simulink model "spwm_three_phase"  (R2020a)
settings: Solver=VariableStepAuto  StartTime=0.0  StopTime=3.0  RelTol=1e-3
values from neighbouring files (symbols this model uses):
  freq_rad = 2*pi*50    (= 314.159265359)    [three_phase_spwm.m]
  Gain = 2000    [three_phase_spwm.m]
  period = 2e-4    (= 0.0002)    [three_phase_spwm.m]
  phase_A = 0    [three_phase_spwm.m]
  phase_B = -2*pi/3    (= -2.09439510239)    [three_phase_spwm.m]
  phase_C = -4*pi/3    (= -4.18879020479)    [three_phase_spwm.m]
  pulse_width = 50    [three_phase_spwm.m]
  T_final_value = 1000    [three_phase_spwm.m]
  T_load_step_time = 1    [three_phase_spwm.m]
  Tz = 1/freq    (= 0.02)    [three_phase_spwm.m]
  Vamp = 1    [three_phase_spwm.m]
  VDC = 400    [three_phase_spwm.m]
  Vpulse = 10    [three_phase_spwm.m]
  Vref = (2/3)*VDC*0.9    (= 240)    [three_phase_spwm.m]
libraries: powerlib x5
settings Model: Creator=Junaed  LastModifiedBy=PC

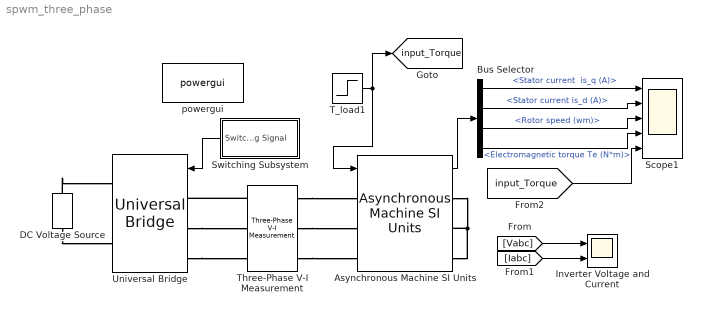
== system spwm_three_phase ==
  Asynchronous Machine SI Units : powerlib/Machines/Asynchronous Machine SI Units  RotorType=Wound  PresetModel=No  MechanicalLoad=Torque Tm  ShowDetailedParameters=on  ReferenceFrame=Rotor  Units=SI  MeasurementBus=off  NominalParameters=[1.845e+04 400 50]  Stator=[0.5968 0.0003495]  Rotor=[0.6258 0.005473]  Cage1=[0.4155 0.002066]  Cage2=[0.4168 0.0003495]  Lm=0.0354  Mechanical=[0.05 0.005879 2]  PolePairs=2  InitialConditions=[1 0 0 0 0 0 0 0]  SimulateSaturation=off  Saturation=[14.03593122, 27.81365428, 53.79336849, 72.68890987, 97.98006896, 148.6815601, 215.7428561, 302.9841135, 428.7778367 ; 230, 322, 414, 460, 506, 552, 598, 644, 690]  LoadFlowParameters=1492000  TsPowergui=0  TsBlock=-1  IterativeModel=Trapezoidal non iterative  IterativeDiscreteModel=Trapezoidal non iterative  Pmec=1.492e+006
  Bus Selector : BusSelector  OutputSignals="Stator measurements.Stator current  is_q (A),Stator measurements.Stator current is_d (A),Mechanical.Rotor speed (wm),Mechanical.Electromagnetic torque Te (N*m)"
  DC Voltage Source : powerlib/Electrical Sources/DC Voltage Source  Amplitude=VDC  Measurements=None
  Inverter Voltage and Current : Scope  NumInputPorts=2
  Scope1 : Scope  NumInputPorts=5
  Switching Subsystem : Subsystem
      settings: PortSchema="{\"entries\":[{\"content\":{\"sides\":[{\"content\":{\"connectorIds\":[\"Out1\"]},\"type\":\"ConnectorPlacement.EquallySpacedRectSide\",\"uuid\":\"666120e6-e3a6-4d41-8608-f47cc973ff78\"},{\"content\":{\"connectorIds\":[],\"side\":\"RIGHT\"},\"type\":\"ConnectorPlacement.EquallySpacedRectSide\",\"uuid\":\"51b09ffb-5a1b-4931-8ff6-f2d904303abf\"},{\"content\":{\"connectorIds\":[],\"side\":\"TOP\"},\"type\":\"ConnectorPlacement.EquallySpacedRectSide\",\"uuid\":\"d8637988-4995-4d87-a31f-ae42bffd7a57\"}]},\"type\":\"ConnectorPlacement.EquallySpacedConnector\",\"uuid\":\"019588fd-0135-4367-b5fb-8d28a8d71eb3\"}],\"packageUris\":[\"http://schema.mathworks.com/mf0/Connector/19700101\"],\"version\":\"1.0\"}"
  T_load1 : Step  Time=T_load_step_time  After=T_final_value  SampleTime=0
  Three-Phase V-I Measurement : powerlib/Measurements/Three-Phase V-I Measurement  VoltageMeasurement=phase-to-phase  SetLabelV=on  LabelV=Vabc  Vpu=off  VpuLL=off  CurrentMeasurement=yes  SetLabelI=on  LabelI=Iabc  Ipu=off  Pbase=100e6  Vbase=500e3  OutputType=Complex  PhasorSimulation=off  PSBequivalent=0
  Universal Bridge : powerlib/Power Electronics/Universal Bridge  Arms=3  SnubberResistance=1e5  SnubberCapacitance=inf  Device=IGBT / Diodes  Ron=1e-3  Lon=0  ForwardVoltages="[  0  0  ]"  ForwardVoltage=0  GTOparameters=[ 10e-6 , 20e-6 ]  IGBTparameters=[ 1e-6 , 2e-6 ]  Measurements=None  Measurements_2=None  converterType=Rectifier
  powergui : powerlib/powergui  Priority=1  SimulationMode=Continuous  SampleTime=50e-6  frequency=60  Iterations=50  frequencyindice=50  Pbase=100e6  ErrMax=1e-4  UnitsV=kV  UnitsW=MW  buscounter=0  FunctionMessages=off  echomessages=off  EnableUseOfTLC=off  CurrentSourceSwitches=off  DisableSnubberDevices=off  DisableRonSwitches=off  DisableVfSwitches=off  DisplayEquations=off  AutomaticDiscreteSolvers=off  SolverType=Tustin/Backward Euler (TBE)  Interpol=off  ExternalGateDelay=off  methode=off  Ts=100  x0status=blocks  SPID=on  SwTol=0  HookPort=off  NonlinearTolerance=1e-4  nMaxIteration=100  ContinueOnMaxIteration=off  RestoreLinks=warning  ResistiveCurrentMeasurement=off  Frange=[0:2:500]  Ylog=off  Xlog=on  ShowGrid=off  save=off  variable=ZData  structure=0  ZoomFFT=off  StartTime=0.0  cycles=1  DisplayStyle=1  fundamental=60  FreqAxis=off  MaxFrequency=1000  frequencyindicesteady=1  RmsSteady=1  display=off
  tag scope: input_Torque=global
  wires:
  T_load1/1 -> Asynchronous Machine SI Units/1, [input_Torque]
  Asynchronous Machine SI Units/1 -> Bus Selector/1
  Bus Selector/1 -> Scope1/1  "<Stator current  is_q (A)>"
  Bus Selector/2 -> Scope1/2  "<Stator current is_d (A)>"
  Bus Selector/3 -> Scope1/3  "<Rotor speed (wm)>"
  Bus Selector/4 -> Scope1/4  "<Electromagnetic torque Te (N*m)>"
  Switching Subsystem/1("Switching Signal ") -> Universal Bridge/1
  [Vabc] -> Inverter Voltage and Current/1
  [Iabc] -> Inverter Voltage and Current/2
  [input_Torque] -> Scope1/5
  connections:
  Asynchronous Machine SI Units/RConn1 -- Asynchronous Machine SI Units/RConn3 -- Asynchronous Machine SI Units/RConn2
  DC Voltage Source/RConn1 -- Universal Bridge/RConn1
  DC Voltage Source/LConn1 -- Universal Bridge/RConn2
  Three-Phase V-I Measurement/LConn1 -- Universal Bridge/LConn1
  Universal Bridge/LConn2 -- Three-Phase V-I Measurement/LConn2
  Universal Bridge/LConn3 -- Three-Phase V-I Measurement/LConn3
  Three-Phase V-I Measurement/RConn1 -- Asynchronous Machine SI Units/LConn1
  Three-Phase V-I Measurement/RConn2 -- Asynchronous Machine SI Units/LConn2
  Three-Phase V-I Measurement/RConn3 -- Asynchronous Machine SI Units/LConn3

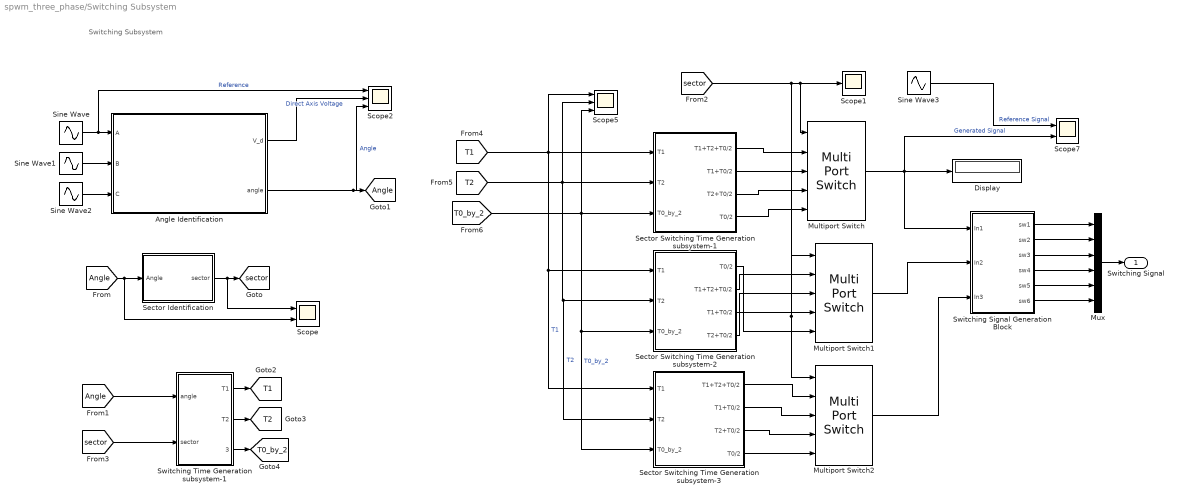
== system spwm_three_phase/Switching Subsystem ==
  note: Switching Subsystem
  Angle Identification : Subsystem
  Display : Display
  Multiport Switch : MultiPortSwitch  DataPortOrder=Specify indices  Inputs=4  DataPortIndices={[1,6],2,5,[3,4]}
  Multiport Switch1 : MultiPortSwitch  DataPortOrder=Specify indices  Inputs=4  DataPortIndices={[2,3],4,1,[5,6]}
  Multiport Switch2 : MultiPortSwitch  DataPortOrder=Specify indices  Inputs=4  DataPortIndices={[4,5],6,3,[1,2]}
  Mux : Mux  Inputs=6
  Scope : Scope  NumInputPorts=2
  Scope1 : Scope
  Scope2 : Scope  NumInputPorts=3
  Scope5 : Scope  NumInputPorts=3
  Scope7 : Scope  NumInputPorts=2
  Sector Identification : Subsystem
  Sector Switching Time Generation subsystem-1 : Subsystem
  Sector Switching Time Generation subsystem-2 : Subsystem
  Sector Switching Time Generation subsystem-3 : Subsystem
  Sine Wave : Sin  Amplitude=Vamp  Frequency=freq_rad  Phase=phase_A  SampleTime=0
  Sine Wave1 : Sin  Amplitude=Vamp  Frequency=freq_rad  Phase=phase_B  SampleTime=0
  Sine Wave2 : Sin  Amplitude=Vamp  Frequency=freq_rad  Phase=phase_C  SampleTime=0
  Sine Wave3 : Sin  Frequency=2*pi*50  SampleTime=0
  Switching Signal Generation Block : Subsystem
  Switching Time Generation subsystem-1 : Subsystem
  "Switching Signal " : Outport
  tag scope: Angle=global, T0_by_2=global, T1=global, T2=global, sector=global
  wires:
  [sector] -> Multiport Switch/1, Scope1/1, Multiport Switch2/1, Multiport Switch1/1
  Multiport Switch/1 -> Scope7/2, Switching Signal Generation Block/1(In1), Display/1  "Generated Signal"
  Angle Identification/2(angle) -> [Angle], Scope2/3  "Angle"
  Sine Wave2/1 -> Angle Identification/3(C)
  Sine Wave1/1 -> Angle Identification/2(B)
  Sine Wave3/1 -> Scope7/1  "Reference Signal"
  [T1] -> Sector Switching Time Generation subsystem-3/1(T1), Sector Switching Time Generation subsystem-2/1(T1), Scope5/1, Sector Switching Time Generation subsystem-1/1(T1)  "T1"
  [T2] -> Sector Switching Time Generation subsystem-3/2(T2), Sector Switching Time Generation subsystem-2/2(T2), Scope5/2, Sector Switching Time Generation subsystem-1/2(T2)  "T2"
  [T0_by_2] -> Sector Switching Time Generation subsystem-2/3(T0_by_2), Sector Switching Time Generation subsystem-3/3(T0_by_2), Scope5/3, Sector Switching Time Generation subsystem-1/3(T0_by_2)  "T0_by_2"
  Sector Switching Time Generation subsystem-1/1(T1+T2+T0/2) -> Multiport Switch/2
  Sector Switching Time Generation subsystem-1/2(T1+T0/2) -> Multiport Switch/3
  Sector Switching Time Generation subsystem-1/3(T2+T0/2) -> Multiport Switch/4
  Sector Switching Time Generation subsystem-1/4(T0/2) -> Multiport Switch/5
  Sector Switching Time Generation subsystem-2/2(T1+T2+T0/2) -> Multiport Switch1/2
  Sector Switching Time Generation subsystem-2/3(T1+T0/2) -> Multiport Switch1/3
  Sector Switching Time Generation subsystem-2/1(T0/2) -> Multiport Switch1/5
  Sector Switching Time Generation subsystem-2/4(T2+T0/2) -> Multiport Switch1/4
  Sector Switching Time Generation subsystem-3/1(T1+T2+T0/2) -> Multiport Switch2/2
  Sector Switching Time Generation subsystem-3/4(T0/2) -> Multiport Switch2/5
  Sector Switching Time Generation subsystem-3/2(T1+T0/2) -> Multiport Switch2/3
  Sector Switching Time Generation subsystem-3/3(T2+T0/2) -> Multiport Switch2/4
  Multiport Switch1/1 -> Switching Signal Generation Block/2(In2)
  Multiport Switch2/1 -> Switching Signal Generation Block/3(In3)
  Angle Identification/1(V_d) -> Scope2/2  "Direct Axis Voltage"
  Sine Wave/1 -> Scope2/1, Angle Identification/1(A)  "Reference"
  Switching Signal Generation Block/1(sw1) -> Mux/1
  Switching Signal Generation Block/2(sw2) -> Mux/2
  Switching Signal Generation Block/3(sw3) -> Mux/3
  Switching Signal Generation Block/4(sw4) -> Mux/4
  Switching Signal Generation Block/5(sw5) -> Mux/5
  Switching Signal Generation Block/6(sw6) -> Mux/6
  Mux/1 -> "Switching Signal "/1
  [Angle] -> Scope/2, Sector Identification/1(Angle)
  Sector Identification/1(sector) -> Scope/1, [sector]
  [sector] -> Switching Time Generation subsystem-1/2(sector)
  [Angle] -> Switching Time Generation subsystem-1/1(angle)
  Switching Time Generation subsystem-1/1(T1) -> [T1]
  Switching Time Generation subsystem-1/2(T2) -> [T2]
  Switching Time Generation subsystem-1/3(T0_by_2) -> [T0_by_2]

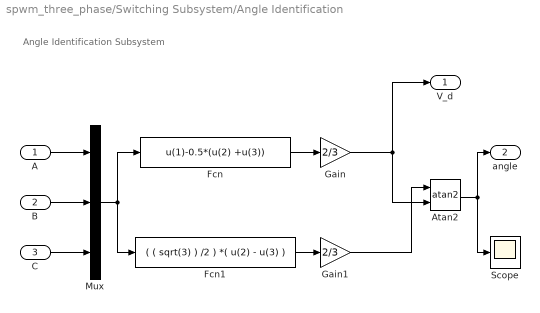
== system spwm_three_phase/Switching Subsystem/Angle Identification ==
  note: Angle Identification Subsystem
  A : Inport
  B : Inport  Port=2
  C : Inport  Port=3
  Atan2 : Trigonometry  Operator=atan2
  Fcn : Fcn  Expr=u(1)-0.5*(u(2) +u(3))
  Fcn1 : Fcn  Expr=( ( sqrt(3) ) /2 ) *( u(2) - u(3) )
  Gain : Gain  Gain=2/3
  Gain1 : Gain  Gain=2/3
  Mux : Mux  Inputs=3
  Scope : Scope
  V_d : Outport
  angle : Outport  Port=2
  wires:
  Fcn1/1 -> Gain1/1
  Gain/1 -> V_d/1, Atan2/2
  Atan2/1 -> Scope/1, angle/1
  Fcn/1 -> Gain/1
  Mux/1 -> Fcn1/1, Fcn/1
  B/1 -> Mux/2
  C/1 -> Mux/3
  Gain1/1 -> Atan2/1
  A/1 -> Mux/1

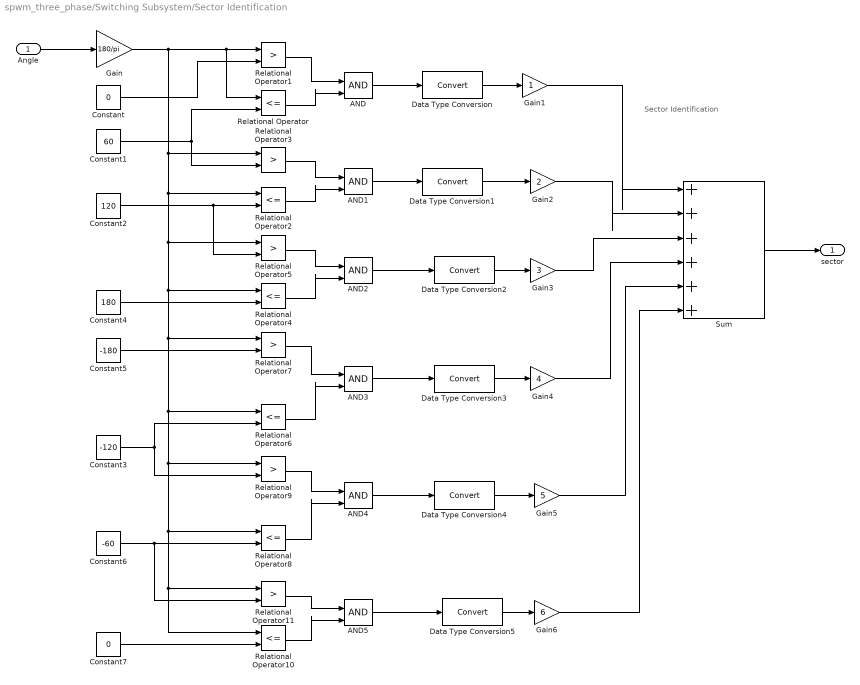
== system spwm_three_phase/Switching Subsystem/Sector Identification ==
  note: Sector Identification
  Angle : Inport
  AND{,1..5} (6 alike) : Logic  IconShape=distinctive  AllPortsSameDT=off  OutDataTypeStr=boolean
  Constant : Constant  Value=0
  Constant1 : Constant  Value=60
  Constant2 : Constant  Value=120
  Constant3 : Constant  Value=-120
  Constant4 : Constant  Value=180
  Constant5 : Constant  Value=-180
  Constant6 : Constant  Value=-60
  Constant7 : Constant  Value=0
  Data Type Conversion{,1..5} (6 alike) : DataTypeConversion
  Gain : Gain  Gain=180/pi
  Gain1 : Gain
  Gain2 : Gain  Gain=2
  Gain3 : Gain  Gain=3
  Gain4 : Gain  Gain=4
  Gain5 : Gain  Gain=5
  Gain6 : Gain  Gain=6
  Relational Operator{,2,4,6,8,10} (6 alike) : RelationalOperator  Operator=<=  OutDataTypeStr=boolean  RndMeth=Simplest
  Relational Operator{1,3,5,7,9,11} (6 alike) : RelationalOperator  Operator=>  OutDataTypeStr=boolean  RndMeth=Simplest
  Sum : Sum  Inputs=|++++++
  sector : Outport
  wires:
  Relational Operator3/1 -> AND1/1
  Gain/1 -> Relational Operator10/1, Relational Operator11/1, Relational Operator8/1, Relational Operator9/1, Relational Operator6/1, Relational Operator7/1, Relational Operator4/1, Relational Operator5/1, Relational Operator2/1, Relational Operator3/1, Relational Operator/1, Relational Operator1/1
  Sum/1 -> sector/1
  Relational Operator1/1 -> AND/1
  Data Type Conversion3/1 -> Gain4/1
  Relational Operator2/1 -> AND1/2
  AND1/1 -> Data Type Conversion1/1
  Relational Operator11/1 -> AND5/1
  Constant6/1 -> Relational Operator11/2, Relational Operator8/2
  Relational Operator5/1 -> AND2/1
  AND/1 -> Data Type Conversion/1
  Constant7/1 -> Relational Operator10/2
  Constant/1 -> Relational Operator1/2
  Constant2/1 -> Relational Operator5/2, Relational Operator2/2
  AND5/1 -> Data Type Conversion5/1
  Relational Operator/1 -> AND/2
  Data Type Conversion5/1 -> Gain6/1
  Constant5/1 -> Relational Operator7/2
  Constant3/1 -> Relational Operator9/2, Relational Operator6/2
  Constant1/1 -> Relational Operator3/2, Relational Operator/2
  Relational Operator10/1 -> AND5/2
  Data Type Conversion1/1 -> Gain2/1
  Angle/1 -> Gain/1
  Data Type Conversion/1 -> Gain1/1
  Relational Operator8/1 -> AND4/2
  Gain4/1 -> Sum/4
  Gain1/1 -> Sum/1
  Data Type Conversion4/1 -> Gain5/1
  Gain3/1 -> Sum/3
  Data Type Conversion2/1 -> Gain3/1
  AND3/1 -> Data Type Conversion3/1
  AND4/1 -> Data Type Conversion4/1
  Constant4/1 -> Relational Operator4/2
  Gain6/1 -> Sum/6
  Relational Operator6/1 -> AND3/2
  Relational Operator9/1 -> AND4/1
  Relational Operator7/1 -> AND3/1
  Relational Operator4/1 -> AND2/2
  AND2/1 -> Data Type Conversion2/1
  Gain5/1 -> Sum/5
  Gain2/1 -> Sum/2

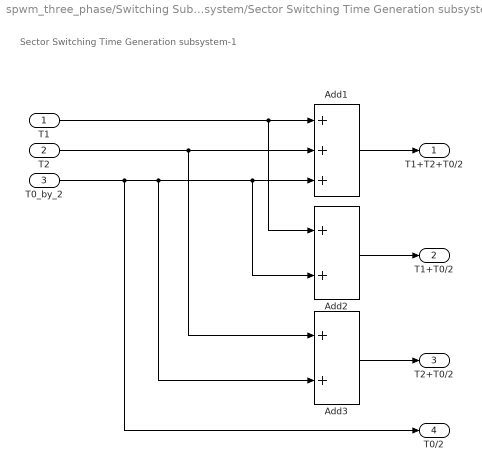
== system spwm_three_phase/Switching Subsystem/Sector Switching Time Generation subsystem-1 ==
  note: Sector Switching Time Generation subsystem-1
  T1 : Inport
  T2 : Inport  Port=2
  T0_by_2 : Inport  Port=3
  Add1 : Sum  Inputs=+++
  Add2 : Sum
  Add3 : Sum
  T1+T2+T0/2 : Outport
  T1+T0/2 : Outport  Port=2
  T2+T0/2 : Outport  Port=3
  T0/2 : Outport  Port=4
  wires:
  Add3/1 -> T2+T0/2/1
  T1/1 -> Add2/1, Add1/1
  Add1/1 -> T1+T2+T0/2/1
  Add2/1 -> T1+T0/2/1
  T0_by_2/1 -> T0/2/1, Add3/2, Add2/2, Add1/3
  T2/1 -> Add3/1, Add1/2

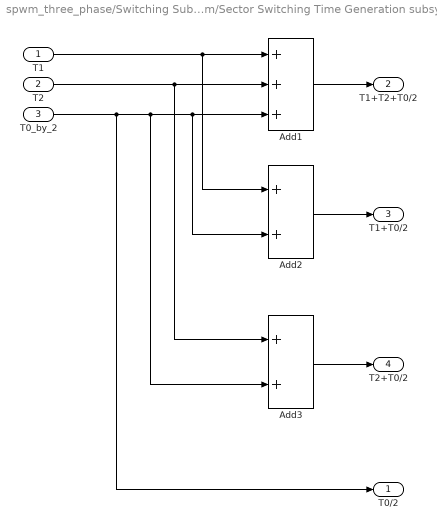
== system spwm_three_phase/Switching Subsystem/Sector Switching Time Generation subsystem-2 ==
  T1 : Inport
  T2 : Inport  Port=2
  T0_by_2 : Inport  Port=3
  Add1 : Sum  Inputs=+++
  Add2 : Sum
  Add3 : Sum
  T0/2 : Outport
  T1+T2+T0/2 : Outport  Port=2
  T1+T0/2 : Outport  Port=3
  T2+T0/2 : Outport  Port=4
  wires:
  T0_by_2/1 -> T0/2/1, Add3/2, Add2/2, Add1/3
  T2/1 -> Add3/1, Add1/2
  Add3/1 -> T2+T0/2/1
  T1/1 -> Add2/1, Add1/1
  Add1/1 -> T1+T2+T0/2/1
  Add2/1 -> T1+T0/2/1

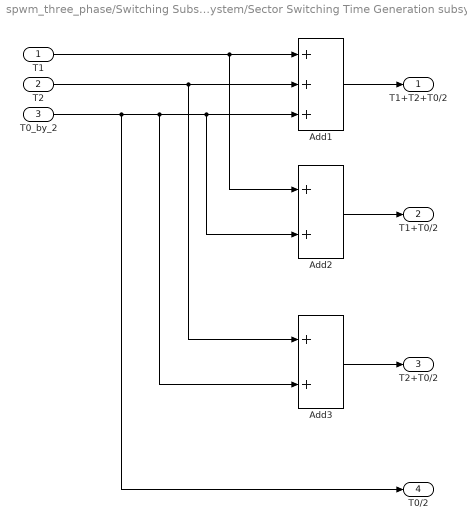
== system spwm_three_phase/Switching Subsystem/Sector Switching Time Generation subsystem-3 ==
  T1 : Inport
  T2 : Inport  Port=2
  T0_by_2 : Inport  Port=3
  Add1 : Sum  Inputs=+++
  Add2 : Sum
  Add3 : Sum
  T1+T2+T0/2 : Outport
  T1+T0/2 : Outport  Port=2
  T2+T0/2 : Outport  Port=3
  T0/2 : Outport  Port=4
  wires:
  T2/1 -> Add3/1, Add1/2
  Add3/1 -> T2+T0/2/1
  T0_by_2/1 -> T0/2/1, Add3/2, Add2/2, Add1/3
  T1/1 -> Add2/1, Add1/1
  Add1/1 -> T1+T2+T0/2/1
  Add2/1 -> T1+T0/2/1

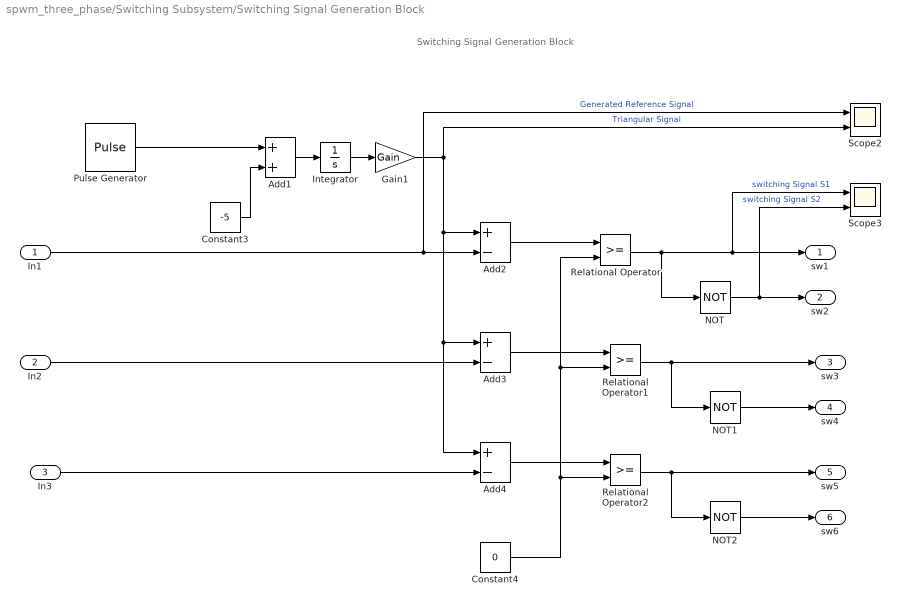
== system spwm_three_phase/Switching Subsystem/Switching Signal Generation Block ==
  note: Switching Signal Generation Block
  In1 : Inport
  In2 : Inport  Port=2
  In3 : Inport  Port=3
  Add1 : Sum
  Add2 : Sum  Inputs=+-
  Add3 : Sum  Inputs=+-
  Add4 : Sum  Inputs=+-
  Constant3 : Constant  Value=-5
  Constant4 : Constant  Value=0
  Gain1 : Gain  Gain=Gain
  Integrator : Integrator
  NOT : Logic  Operator=NOT  IconShape=distinctive  AllPortsSameDT=off  OutDataTypeStr=boolean
  NOT1 : Logic  Operator=NOT  IconShape=distinctive  AllPortsSameDT=off  OutDataTypeStr=boolean
  NOT2 : Logic  Operator=NOT  IconShape=distinctive  AllPortsSameDT=off  OutDataTypeStr=boolean
  Pulse Generator : DiscretePulseGenerator  PulseType=Time based  Amplitude=Vpulse  Period=period  PulseWidth=pulse_width
  Relational Operator : RelationalOperator  OutDataTypeStr=boolean  ZeroCross=off  RndMeth=Simplest
  Relational Operator1 : RelationalOperator  OutDataTypeStr=boolean  ZeroCross=off  RndMeth=Simplest
  Relational Operator2 : RelationalOperator  OutDataTypeStr=boolean  ZeroCross=off  RndMeth=Simplest
  Scope2 : Scope  NumInputPorts=2
  Scope3 : Scope  NumInputPorts=2
  sw1 : Outport
  sw2 : Outport  Port=2
  sw3 : Outport  Port=3
  sw4 : Outport  Port=4
  sw5 : Outport  Port=5
  sw6 : Outport  Port=6
  wires:
  Add4/1 -> Relational Operator2/1
  Pulse Generator/1 -> Add1/1
  Relational Operator/1 -> sw1/1, Scope3/1, NOT/1  "switching Signal S1"
  Relational Operator2/1 -> sw5/1, NOT2/1
  Gain1/1 -> Scope2/2, Add3/1, Add4/1, Add2/1  "Triangular Signal"
  Relational Operator1/1 -> sw3/1, NOT1/1
  NOT2/1 -> sw6/1
  Integrator/1 -> Gain1/1
  Add1/1 -> Integrator/1
  In1/1 -> Scope2/1, Add2/2  "Generated Reference Signal"
  Constant3/1 -> Add1/2
  Add3/1 -> Relational Operator1/1
  NOT/1 -> sw2/1, Scope3/2  "switching Signal S2"
  Add2/1 -> Relational Operator/1
  NOT1/1 -> sw4/1
  Constant4/1 -> Relational Operator/2, Relational Operator1/2, Relational Operator2/2
  In3/1 -> Add4/2
  In2/1 -> Add3/2

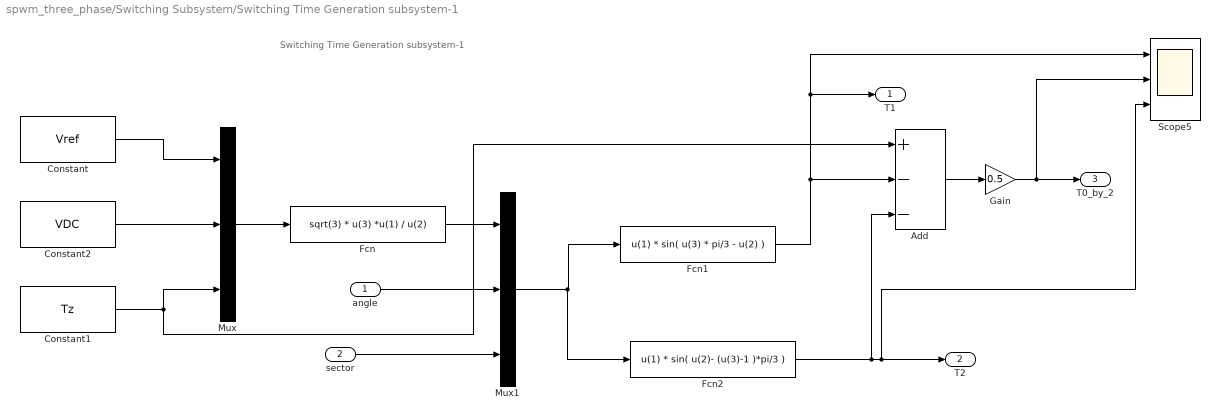
== system spwm_three_phase/Switching Subsystem/Switching Time Generation subsystem-1 ==
  note: Switching Time Generation subsystem-1
  angle : Inport
  sector : Inport  Port=2
  Add : Sum  Inputs=+--
  Constant : Constant  Value=Vref
  Constant1 : Constant  Value=Tz
  Constant2 : Constant  Value=VDC
  Fcn : Fcn  Expr=sqrt(3) * u(3) *u(1) / u(2)
  Fcn1 : Fcn  Expr=u(1) * sin( u(3) * pi/3 - u(2) )
  Fcn2 : Fcn  Expr=u(1) * sin( u(2)- (u(3)-1 )*pi/3 )
  Gain : Gain  Gain=0.5
  Mux : Mux  Inputs=3
  Mux1 : Mux  Inputs=3
  Scope5 : Scope  NumInputPorts=3
  T1 : Outport
  T2 : Outport  Port=2
  T0_by_2 : Outport  Port=3
  wires:
  Add/1 -> Gain/1
  sector/1 -> Mux1/3
  Mux1/1 -> Fcn2/1, Fcn1/1
  Constant/1 -> Mux/1
  Fcn2/1 -> T2/1, Scope5/3, Add/3
  Fcn1/1 -> T1/1, Scope5/1, Add/2
  Gain/1 -> Scope5/2, T0_by_2/1
  Constant2/1 -> Mux/2
  Fcn/1 -> Mux1/1
  Constant1/1 -> Mux/3, Add/1
  Mux/1 -> Fcn/1
  angle/1 -> Mux1/2
